simulink model "windTurbine_th"  (R2018b)
settings: Solver=VariableStepAuto  StartTime=0.0  StopTime=100  RelTol=1e-3
libraries: windTurbine_ul x1
settings Model: Creator=asiddiq2  LastModifiedBy=asiddiq2

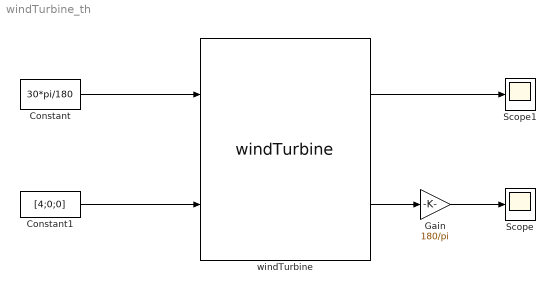
== system windTurbine_th ==
  Constant : Constant  Value=30*pi/180  VectorParams1D=off
  Constant1 : Constant  Value=[4;0;0]  VectorParams1D=off
  Gain : Gain  Gain=180/pi
  Scope : Scope
  Scope1 : Scope
  windTurbine : windTurbine_ul/windTurbine  Cp=0.6  rhoFluid=1  diam=1  dampCoeff=1.5  Izz=10  iniYaw=0  Kp=0.5  Ki=0  Kd=4  tau=0.5
  wires:
  Constant/1 -> windTurbine/1
  Constant1/1 -> windTurbine/2
  windTurbine/1 -> Scope1/1
  windTurbine/2 -> Gain/1
  Gain/1 -> Scope/1
